simulink model "MVS_Dynamic_Trigger_Two_Layers_NoRA"  (R2024a)
settings: Solver=ode5  StartTime=0.0  StopTime=180  FixedStep=0.01  RelTol=1e-3
(part 2 of 4)

== system MVS_Dynamic_Trigger_Two_Layers_NoRA/High-Level Agent 1/Trajectory Planner ==
  e_tilde_xi : Inport
  e_tilde_vi : Inport  Port=2
  delta_xi : Inport  Port=3
  delta_vi : Inport  Port=4
  acc_ref : Inport  Port=5
  states_high : Inport  Port=6
  states_low : Inport  Port=7
  Achievability assurance : Subsystem
  Cooperative tracking : Subsystem
  Input compensator : MATLAB Function  TreatAsAtomicUnit=on
  State select : MATLAB Function  TreatAsAtomicUnit=on
  u_i : Outport
  wires:
  e_tilde_xi/1 -> Cooperative tracking/1(e_tilde_xi)
  e_tilde_vi/1 -> Cooperative tracking/2(e_tilde_vi)
  delta_xi/1 -> Cooperative tracking/3(delta_xi)
  delta_vi/1 -> Cooperative tracking/4(delta_vi)
  acc_ref/1 -> Cooperative tracking/5(acc_ref)
  Input compensator/1(u_i) -> u_i/1
  states_high/1 -> State select/1(states_high)
  states_low/1 -> State select/2(states_low)
  State select/1(v_i) -> Achievability assurance/1(v_i), Cooperative tracking/6(v_i)
  State select/2(delta_x_tilde) -> Achievability assurance/2(delta_x)
  State select/3(delta_v_tilde) -> Achievability assurance/3(delta_v)
  State select/4(a_d) -> Achievability assurance/4(a_d)
  Cooperative tracking/1(u_i_track) -> Input compensator/1(u_i_track)
  Achievability assurance/1(u_i_restrict) -> Input compensator/2(u_i_restrict)
  Achievability assurance/2(delta_low_norm) -> Input compensator/3(delta_low_norm)

== system MVS_Dynamic_Trigger_Two_Layers_NoRA/High-Level Agent 2/High-Level Dynamics ==
  u_i : Inport
  Memory : Memory  InitialCondition=zeros(3,1)
  Position : Integrator  InitialCondition=ini_pos
  Saturation_acc : Saturate  UpperLimit=acc_up_limit  LowerLimit=acc_low_limit
  Saturation_vel : Saturate  UpperLimit=vel_up_limit  LowerLimit=vel_low_limit
  Speed : Integrator  InitialCondition=[0;0;0]
  v_2 : Scope
  x_2 : Scope
  x_i : Outport
  v_i : Outport  Port=2
  a_i : Outport  Port=3
  wires:
  Position/1 -> x_i/1, x_2/1
  u_i/1 -> Memory/1
  Saturation_acc/1 -> a_i/1, Speed/1
  Speed/1 -> v_2/1, Saturation_vel/1
  Saturation_vel/1 -> v_i/1, Position/1
  Memory/1 -> Saturation_acc/1

== system MVS_Dynamic_Trigger_Two_Layers_NoRA/High-Level Agent 2/Trajectory Planner ==
  e_tilde_xi : Inport
  e_tilde_vi : Inport  Port=2
  delta_xi : Inport  Port=3
  delta_vi : Inport  Port=4
  acc_ref : Inport  Port=5
  states_high : Inport  Port=6
  states_low : Inport  Port=7
  Achievability assurance : Subsystem
  Cooperative tracking : Subsystem
  Input compensator : MATLAB Function  TreatAsAtomicUnit=on
  State select : MATLAB Function  TreatAsAtomicUnit=on
  u_i : Outport
  wires:
  e_tilde_xi/1 -> Cooperative tracking/1(e_tilde_xi)
  e_tilde_vi/1 -> Cooperative tracking/2(e_tilde_vi)
  delta_xi/1 -> Cooperative tracking/3(delta_xi)
  delta_vi/1 -> Cooperative tracking/4(delta_vi)
  acc_ref/1 -> Cooperative tracking/5(acc_ref)
  Input compensator/1(u_i) -> u_i/1
  states_high/1 -> State select/1(states_high)
  states_low/1 -> State select/2(states_low)
  State select/1(v_i) -> Achievability assurance/1(v_i), Cooperative tracking/6(v_i)
  State select/2(delta_x_tilde) -> Achievability assurance/2(delta_x)
  State select/3(delta_v_tilde) -> Achievability assurance/3(delta_v)
  State select/4(a_d) -> Achievability assurance/4(a_d)
  Cooperative tracking/1(u_i_track) -> Input compensator/1(u_i_track)
  Achievability assurance/1(u_i_restrict) -> Input compensator/2(u_i_restrict)
  Achievability assurance/2(delta_low_norm) -> Input compensator/3(delta_low_norm)

== system MVS_Dynamic_Trigger_Two_Layers_NoRA/High-Level Agent 3/High-Level Dynamics ==
  u_i : Inport
  Memory : Memory  InitialCondition=zeros(3,1)
  Position : Integrator  InitialCondition=ini_pos
  Saturation_acc : Saturate  UpperLimit=acc_up_limit  LowerLimit=acc_low_limit
  Saturation_vel : Saturate  UpperLimit=vel_up_limit  LowerLimit=vel_low_limit
  Speed : Integrator  InitialCondition=[0;0;0]
  v_3 : Scope
  x_3 : Scope
  x_i : Outport
  v_i : Outport  Port=2
  a_i : Outport  Port=3
  wires:
  Position/1 -> x_i/1, x_3/1
  u_i/1 -> Memory/1
  Saturation_acc/1 -> a_i/1, Speed/1
  Speed/1 -> v_3/1, Saturation_vel/1
  Saturation_vel/1 -> v_i/1, Position/1
  Memory/1 -> Saturation_acc/1

== system MVS_Dynamic_Trigger_Two_Layers_NoRA/High-Level Agent 3/Trajectory Planner ==
  e_tilde_xi : Inport
  e_tilde_vi : Inport  Port=2
  delta_xi : Inport  Port=3
  delta_vi : Inport  Port=4
  acc_ref : Inport  Port=5
  states_high : Inport  Port=6
  states_low : Inport  Port=7
  Achievability assurance : Subsystem
  Cooperative tracking : Subsystem
  Input compensator : MATLAB Function  TreatAsAtomicUnit=on
  State select : MATLAB Function  TreatAsAtomicUnit=on
  u_i : Outport
  wires:
  e_tilde_xi/1 -> Cooperative tracking/1(e_tilde_xi)
  e_tilde_vi/1 -> Cooperative tracking/2(e_tilde_vi)
  delta_xi/1 -> Cooperative tracking/3(delta_xi)
  delta_vi/1 -> Cooperative tracking/4(delta_vi)
  acc_ref/1 -> Cooperative tracking/5(acc_ref)
  Input compensator/1(u_i) -> u_i/1
  states_high/1 -> State select/1(states_high)
  states_low/1 -> State select/2(states_low)
  State select/1(v_i) -> Achievability assurance/1(v_i), Cooperative tracking/6(v_i)
  State select/2(delta_x_tilde) -> Achievability assurance/2(delta_x)
  State select/3(delta_v_tilde) -> Achievability assurance/3(delta_v)
  State select/4(a_d) -> Achievability assurance/4(a_d)
  Cooperative tracking/1(u_i_track) -> Input compensator/1(u_i_track)
  Achievability assurance/1(u_i_restrict) -> Input compensator/2(u_i_restrict)
  Achievability assurance/2(delta_low_norm) -> Input compensator/3(delta_low_norm)

== system MVS_Dynamic_Trigger_Two_Layers_NoRA/High-Level Agent 4/High-Level Dynamics ==
  u_i : Inport
  Memory : Memory  InitialCondition=zeros(3,1)
  Position : Integrator  InitialCondition=ini_pos
  Saturation_acc : Saturate  UpperLimit=acc_up_limit  LowerLimit=acc_low_limit
  Saturation_vel : Saturate  UpperLimit=vel_up_limit  LowerLimit=vel_low_limit
  Speed : Integrator  InitialCondition=[0;0;0]
  v_4 : Scope
  x_4 : Scope
  x_i : Outport
  v_i : Outport  Port=2
  a_i : Outport  Port=3
  wires:
  Position/1 -> x_i/1, x_4/1
  u_i/1 -> Memory/1
  Saturation_acc/1 -> a_i/1, Speed/1
  Speed/1 -> v_4/1, Saturation_vel/1
  Saturation_vel/1 -> v_i/1, Position/1
  Memory/1 -> Saturation_acc/1

== system MVS_Dynamic_Trigger_Two_Layers_NoRA/High-Level Agent 4/Trajectory Planner ==
  e_tilde_xi : Inport
  e_tilde_vi : Inport  Port=2
  delta_xi : Inport  Port=3
  delta_vi : Inport  Port=4
  acc_ref : Inport  Port=5
  states_high : Inport  Port=6
  states_low : Inport  Port=7
  Achievability assurance : Subsystem
  Cooperative tracking : Subsystem
  Input compensator : MATLAB Function  TreatAsAtomicUnit=on
  State select : MATLAB Function  TreatAsAtomicUnit=on
  u_i : Outport
  wires:
  e_tilde_xi/1 -> Cooperative tracking/1(e_tilde_xi)
  e_tilde_vi/1 -> Cooperative tracking/2(e_tilde_vi)
  delta_xi/1 -> Cooperative tracking/3(delta_xi)
  delta_vi/1 -> Cooperative tracking/4(delta_vi)
  acc_ref/1 -> Cooperative tracking/5(acc_ref)
  Input compensator/1(u_i) -> u_i/1
  states_high/1 -> State select/1(states_high)
  states_low/1 -> State select/2(states_low)
  State select/1(v_i) -> Achievability assurance/1(v_i), Cooperative tracking/6(v_i)
  State select/2(delta_x_tilde) -> Achievability assurance/2(delta_x)
  State select/3(delta_v_tilde) -> Achievability assurance/3(delta_v)
  State select/4(a_d) -> Achievability assurance/4(a_d)
  Cooperative tracking/1(u_i_track) -> Input compensator/1(u_i_track)
  Achievability assurance/1(u_i_restrict) -> Input compensator/2(u_i_restrict)
  Achievability assurance/2(delta_low_norm) -> Input compensator/3(delta_low_norm)

== system MVS_Dynamic_Trigger_Two_Layers_NoRA/High-Level Agent 5/High-Level Dynamics ==
  u_i : Inport
  Memory : Memory  InitialCondition=zeros(3,1)
  Position : Integrator  InitialCondition=ini_pos
  Saturation_acc : Saturate  UpperLimit=acc_up_limit  LowerLimit=acc_low_limit
  Saturation_vel : Saturate  UpperLimit=vel_up_limit  LowerLimit=vel_low_limit
  Speed : Integrator  InitialCondition=[0;0;0]
  v_5 : Scope
  x_5 : Scope
  x_i : Outport
  v_i : Outport  Port=2
  a_i : Outport  Port=3
  wires:
  Position/1 -> x_i/1, x_5/1
  u_i/1 -> Memory/1
  Saturation_acc/1 -> a_i/1, Speed/1
  Speed/1 -> v_5/1, Saturation_vel/1
  Saturation_vel/1 -> v_i/1, Position/1
  Memory/1 -> Saturation_acc/1

== system MVS_Dynamic_Trigger_Two_Layers_NoRA/High-Level Agent 5/Trajectory Planner ==
  e_tilde_xi : Inport
  e_tilde_vi : Inport  Port=2
  delta_xi : Inport  Port=3
  delta_vi : Inport  Port=4
  acc_ref : Inport  Port=5
  states_high : Inport  Port=6
  states_low : Inport  Port=7
  Achievability assurance : Subsystem
  Cooperative tracking : Subsystem
  Input compensator : MATLAB Function  TreatAsAtomicUnit=on
  State select : MATLAB Function  TreatAsAtomicUnit=on
  u_i : Outport
  wires:
  e_tilde_xi/1 -> Cooperative tracking/1(e_tilde_xi)
  e_tilde_vi/1 -> Cooperative tracking/2(e_tilde_vi)
  delta_xi/1 -> Cooperative tracking/3(delta_xi)
  delta_vi/1 -> Cooperative tracking/4(delta_vi)
  acc_ref/1 -> Cooperative tracking/5(acc_ref)
  Input compensator/1(u_i) -> u_i/1
  states_high/1 -> State select/1(states_high)
  states_low/1 -> State select/2(states_low)
  State select/1(v_i) -> Achievability assurance/1(v_i), Cooperative tracking/6(v_i)
  State select/2(delta_x_tilde) -> Achievability assurance/2(delta_x)
  State select/3(delta_v_tilde) -> Achievability assurance/3(delta_v)
  State select/4(a_d) -> Achievability assurance/4(a_d)
  Cooperative tracking/1(u_i_track) -> Input compensator/1(u_i_track)
  Achievability assurance/1(u_i_restrict) -> Input compensator/2(u_i_restrict)
  Achievability assurance/2(delta_low_norm) -> Input compensator/3(delta_low_norm)

== system MVS_Dynamic_Trigger_Two_Layers_NoRA/High-Level Agent 6/High-Level Dynamics ==
  u_i : Inport
  Memory : Memory  InitialCondition=zeros(3,1)
  Position : Integrator  InitialCondition=ini_pos
  Saturation_acc : Saturate  UpperLimit=acc_up_limit  LowerLimit=acc_low_limit
  Saturation_vel : Saturate  UpperLimit=vel_up_limit  LowerLimit=vel_low_limit
  Speed : Integrator  InitialCondition=[0;0;0]
  v_6 : Scope
  x_6 : Scope
  x_i : Outport
  v_i : Outport  Port=2
  a_i : Outport  Port=3
  wires:
  Position/1 -> x_i/1, x_6/1
  u_i/1 -> Memory/1
  Saturation_acc/1 -> a_i/1, Speed/1
  Speed/1 -> v_6/1, Saturation_vel/1
  Saturation_vel/1 -> v_i/1, Position/1
  Memory/1 -> Saturation_acc/1

== system MVS_Dynamic_Trigger_Two_Layers_NoRA/High-Level Agent 6/Trajectory Planner ==
  e_tilde_xi : Inport
  e_tilde_vi : Inport  Port=2
  delta_xi : Inport  Port=3
  delta_vi : Inport  Port=4
  acc_ref : Inport  Port=5
  states_high : Inport  Port=6
  states_low : Inport  Port=7
  Achievability assurance : Subsystem
  Cooperative tracking : Subsystem
  Input compensator : MATLAB Function  TreatAsAtomicUnit=on
  State select : MATLAB Function  TreatAsAtomicUnit=on
  u_i : Outport
  wires:
  e_tilde_xi/1 -> Cooperative tracking/1(e_tilde_xi)
  e_tilde_vi/1 -> Cooperative tracking/2(e_tilde_vi)
  delta_xi/1 -> Cooperative tracking/3(delta_xi)
  delta_vi/1 -> Cooperative tracking/4(delta_vi)
  acc_ref/1 -> Cooperative tracking/5(acc_ref)
  Input compensator/1(u_i) -> u_i/1
  states_high/1 -> State select/1(states_high)
  states_low/1 -> State select/2(states_low)
  State select/1(v_i) -> Achievability assurance/1(v_i), Cooperative tracking/6(v_i)
  State select/2(delta_x_tilde) -> Achievability assurance/2(delta_x)
  State select/3(delta_v_tilde) -> Achievability assurance/3(delta_v)
  State select/4(a_d) -> Achievability assurance/4(a_d)
  Cooperative tracking/1(u_i_track) -> Input compensator/1(u_i_track)
  Achievability assurance/1(u_i_restrict) -> Input compensator/2(u_i_restrict)
  Achievability assurance/2(delta_low_norm) -> Input compensator/3(delta_low_norm)

== system MVS_Dynamic_Trigger_Two_Layers_NoRA/UGV 1/Kinematics controller ==
  global_ref : Inport
  global_current_state : Inport  Port=2
  Body error : Scope
  Bus Creator : BusCreator  Inputs=2
  Clock : Clock
  Error calculation : MATLAB Function  TreatAsAtomicUnit=on
  Global error : Scope
  Saturation : Saturate  UpperLimit=[7; tan(2/9 * pi)]  LowerLimit=-[7; tan(2/9 * pi)]
  Control input : Outport
  wires:
  Bus Creator/1 -> Saturation/1
  Error calculation/1(vel_rear) -> Bus Creator/1
  global_ref/1 -> Error calculation/1(ref_3d)
  global_current_state/1 -> Error calculation/2(pos_bike)
  Error calculation/2(tan_sigma) -> Bus Creator/2
  Saturation/1 -> Control input/1
  Error calculation/3(pos_error_global) -> Global error/1
  Error calculation/4(pos_error_body) -> Body error/1
  Clock/1 -> Error calculation/3(t)

== system MVS_Dynamic_Trigger_Two_Layers_NoRA/UGV 2/Kinematics controller ==
  global_ref : Inport
  global_current_state : Inport  Port=2
  Body error : Scope
  Bus Creator : BusCreator  Inputs=2
  Clock : Clock
  Error calculation : MATLAB Function  TreatAsAtomicUnit=on
  Global error : Scope
  Saturation : Saturate  UpperLimit=[7; tan(2/9 * pi)]  LowerLimit=-[7; tan(2/9 * pi)]
  Control input : Outport
  wires:
  Bus Creator/1 -> Saturation/1
  Error calculation/1(vel_rear) -> Bus Creator/1
  global_ref/1 -> Error calculation/1(ref_3d)
  global_current_state/1 -> Error calculation/2(pos_bike)
  Error calculation/2(tan_sigma) -> Bus Creator/2
  Saturation/1 -> Control input/1
  Error calculation/3(pos_error_global) -> Global error/1
  Error calculation/4(pos_error_body) -> Body error/1
  Clock/1 -> Error calculation/3(t)

== system MVS_Dynamic_Trigger_Two_Layers_NoRA/UGV 3/Kinematics controller ==
  global_ref : Inport
  global_current_state : Inport  Port=2
  Body error : Scope
  Bus Creator : BusCreator  Inputs=2
  Error calculation : MATLAB Function  TreatAsAtomicUnit=on
  Global error : Scope
  Saturation : Saturate  UpperLimit=[7; tan(2/9 * pi)]  LowerLimit=-[7; tan(2/9 * pi)]
  Control input : Outport
  wires:
  Bus Creator/1 -> Saturation/1
  Error calculation/1(vel_rear) -> Bus Creator/1
  global_ref/1 -> Error calculation/1(ref_3d)
  global_current_state/1 -> Error calculation/2(pos_bike)
  Error calculation/2(tan_sigma) -> Bus Creator/2
  Saturation/1 -> Control input/1
  Error calculation/3(pos_error_global) -> Global error/1
  Error calculation/4(pos_error_body) -> Body error/1

== system MVS_Dynamic_Trigger_Two_Layers_NoRA/UGV 4/Kinematics controller ==
  global_ref : Inport
  global_current_state : Inport  Port=2
  Body error : Scope
  Bus Creator : BusCreator  Inputs=2
  Error calculation : MATLAB Function  TreatAsAtomicUnit=on
  Global error : Scope
  Saturation : Saturate  UpperLimit=[7; tan(2/9 * pi)]  LowerLimit=-[7; tan(2/9 * pi)]
  Control input : Outport
  wires:
  Bus Creator/1 -> Saturation/1
  Error calculation/1(vel_rear) -> Bus Creator/1
  global_ref/1 -> Error calculation/1(ref_3d)
  global_current_state/1 -> Error calculation/2(pos_bike)
  Error calculation/2(tan_sigma) -> Bus Creator/2
  Saturation/1 -> Control input/1
  Error calculation/3(pos_error_global) -> Global error/1
  Error calculation/4(pos_error_body) -> Body error/1

== system MVS_Dynamic_Trigger_Two_Layers_NoRA/Communication Preparation 1/Reference Filter/Adaptive filter ==
  pos_ref : Inport
  vel_ref : Inport  Port=2
  current_pos : Inport  Port=3
  Filter error 1 : Scope
  Input compensator : MATLAB Function  TreatAsAtomicUnit=on
  Integrator : Integrator  InitialCondition=[0;0;0]
  Nominal filter : MATLAB Function  TreatAsAtomicUnit=on
  Scope : Scope
  u_i : Outport
  filter_error : Outport  Port=2
  wires:
  current_pos/1 -> Nominal filter/3(current_pos)
  vel_ref/1 -> Nominal filter/2(vel_ref)
  pos_ref/1 -> Nominal filter/1(pos_ref)
  Nominal filter/1(u_i_nom) -> Input compensator/1(u_i_nom)
  Input compensator/2(Xi_i_dot) -> Integrator/1
  Integrator/1 -> Scope/1, Input compensator/2(Xi_i)
  Input compensator/1(u_i) -> u_i/1
  Nominal filter/2(filter_error) -> filter_error/1, Filter error 1/1

== system MVS_Dynamic_Trigger_Two_Layers_NoRA/Communication Preparation 2/Reference Filter/Adaptive filter ==
  pos_ref : Inport
  vel_ref : Inport  Port=2
  current_pos : Inport  Port=3
  Filter error 2 : Scope
  Input compensator : MATLAB Function  TreatAsAtomicUnit=on
  Integrator : Integrator  InitialCondition=[0;0;0]
  Nominal filter : MATLAB Function  TreatAsAtomicUnit=on
  Xi_filter_2 : Scope
  u_i : Outport
  filter_error : Outport  Port=2
  wires:
  current_pos/1 -> Nominal filter/3(current_pos)
  vel_ref/1 -> Nominal filter/2(vel_ref)
  pos_ref/1 -> Nominal filter/1(pos_ref)
  Nominal filter/1(u_i_nom) -> Input compensator/1(u_i_nom)
  Input compensator/2(Xi_i_dot) -> Integrator/1
  Integrator/1 -> Xi_filter_2/1, Input compensator/2(Xi_i)
  Input compensator/1(u_i) -> u_i/1
  Nominal filter/2(filter_error) -> filter_error/1, Filter error 2/1

== system MVS_Dynamic_Trigger_Two_Layers_NoRA/Communication Preparation 3/Reference Filter/Adaptive filter ==
  pos_ref : Inport
  vel_ref : Inport  Port=2
  current_pos : Inport  Port=3
  Filter error 3 : Scope
  Input compensator : MATLAB Function  TreatAsAtomicUnit=on
  Integrator : Integrator  InitialCondition=[0;0;0]
  Nominal filter : MATLAB Function  TreatAsAtomicUnit=on
  Xi_filter_3 : Scope
  u_i : Outport
  filter_error : Outport  Port=2
  wires:
  current_pos/1 -> Nominal filter/3(current_pos)
  vel_ref/1 -> Nominal filter/2(vel_ref)
  pos_ref/1 -> Nominal filter/1(pos_ref)
  Nominal filter/1(u_i_nom) -> Input compensator/1(u_i_nom)
  Input compensator/2(Xi_i_dot) -> Integrator/1
  Integrator/1 -> Xi_filter_3/1, Input compensator/2(Xi_i)
  Input compensator/1(u_i) -> u_i/1
  Nominal filter/2(filter_error) -> filter_error/1, Filter error 3/1

== system MVS_Dynamic_Trigger_Two_Layers_NoRA/Communication Preparation 4/Reference Filter/Adaptive filter ==
  pos_ref : Inport
  vel_ref : Inport  Port=2
  current_pos : Inport  Port=3
  Filter error 4 : Scope
  Input compensator : MATLAB Function  TreatAsAtomicUnit=on
  Integrator : Integrator  InitialCondition=[0;0;0]
  Nominal filter : MATLAB Function  TreatAsAtomicUnit=on
  Xi_filter_4 : Scope
  u_i : Outport
  filter_error : Outport  Port=2
  wires:
  current_pos/1 -> Nominal filter/3(current_pos)
  vel_ref/1 -> Nominal filter/2(vel_ref)
  pos_ref/1 -> Nominal filter/1(pos_ref)
  Nominal filter/1(u_i_nom) -> Input compensator/1(u_i_nom)
  Input compensator/2(Xi_i_dot) -> Integrator/1
  Integrator/1 -> Xi_filter_4/1, Input compensator/2(Xi_i)
  Input compensator/1(u_i) -> u_i/1
  Nominal filter/2(filter_error) -> filter_error/1, Filter error 4/1

== system MVS_Dynamic_Trigger_Two_Layers_NoRA/Communication Preparation 5/Reference Filter/Adaptive filter ==
  pos_ref : Inport
  vel_ref : Inport  Port=2
  current_pos : Inport  Port=3
  Filter error 5 : Scope
  Input compensator : MATLAB Function  TreatAsAtomicUnit=on
  Integrator : Integrator  InitialCondition=[0;0;0]
  Nominal filter : MATLAB Function  TreatAsAtomicUnit=on
  Xi_filter_5 : Scope
  u_i : Outport
  filter_error : Outport  Port=2
  wires:
  current_pos/1 -> Nominal filter/3(current_pos)
  vel_ref/1 -> Nominal filter/2(vel_ref)
  pos_ref/1 -> Nominal filter/1(pos_ref)
  Nominal filter/1(u_i_nom) -> Input compensator/1(u_i_nom)
  Input compensator/2(Xi_i_dot) -> Integrator/1
  Integrator/1 -> Xi_filter_5/1, Input compensator/2(Xi_i)
  Input compensator/1(u_i) -> u_i/1
  Nominal filter/2(filter_error) -> filter_error/1, Filter error 5/1

== system MVS_Dynamic_Trigger_Two_Layers_NoRA/Communication Preparation 6/Reference Filter/Adaptive filter ==
  pos_ref : Inport
  vel_ref : Inport  Port=2
  current_pos : Inport  Port=3
  Filter error 6 : Scope
  Input compensator : MATLAB Function  TreatAsAtomicUnit=on
  Integrator : Integrator  InitialCondition=[0;0;0]
  Nominal filter : MATLAB Function  TreatAsAtomicUnit=on
  Xi_filter_6 : Scope
  u_i : Outport
  filter_error : Outport  Port=2
  wires:
  current_pos/1 -> Nominal filter/3(current_pos)
  vel_ref/1 -> Nominal filter/2(vel_ref)
  pos_ref/1 -> Nominal filter/1(pos_ref)
  Nominal filter/1(u_i_nom) -> Input compensator/1(u_i_nom)
  Input compensator/2(Xi_i_dot) -> Integrator/1
  Integrator/1 -> Xi_filter_6/1, Input compensator/2(Xi_i)
  Input compensator/1(u_i) -> u_i/1
  Nominal filter/2(filter_error) -> filter_error/1, Filter error 6/1

== system MVS_Dynamic_Trigger_Two_Layers_NoRA/High-Level Agent 1/Trajectory Planner/Achievability assurance ==
  v_i : Inport
  delta_x : Inport  Port=2
  delta_v : Inport  Port=3
  a_d : Inport  Port=4
  Input compensator : MATLAB Function  TreatAsAtomicUnit=on
  Integrator : Integrator  InitialCondition=[0;0;0]
  Nominal SMC : MATLAB Function  TreatAsAtomicUnit=on
  low_error_norm_1 : Scope
  u_i_res : Scope
  u_i_restrict : Outport
  delta_low_norm : Outport  Port=2
  wires:
  delta_x/1 -> Nominal SMC/1(delta_x)
  delta_v/1 -> Nominal SMC/2(delta_v)
  a_d/1 -> Nominal SMC/3(a_d)
  Nominal SMC/2(delta_norm) -> delta_low_norm/1, low_error_norm_1/1
  Integrator/1 -> Input compensator/3(Xi_i)
  Input compensator/2(Xi_i_dot) -> Integrator/1
  Input compensator/1(u_i_actual) -> u_i_res/1, u_i_restrict/1
  v_i/1 -> Input compensator/2(v_i)
  Nominal SMC/1(u_restrict) -> Input compensator/1(u_i_restrict)

== system MVS_Dynamic_Trigger_Two_Layers_NoRA/High-Level Agent 1/Trajectory Planner/Cooperative tracking ==
  e_tilde_xi : Inport
  e_tilde_vi : Inport  Port=2
  delta_xi : Inport  Port=3
  delta_vi : Inport  Port=4
  acc_ref : Inport  Port=5
  v_i : Inport  Port=6
  Input compensator : MATLAB Function  TreatAsAtomicUnit=on
  Integrator : Integrator  InitialCondition=[0;0;0]
  Nominal sliding mode controller : MATLAB Function  TreatAsAtomicUnit=on
  u_i_tra : Scope
  u_i_track : Outport
  wires:
  acc_ref/1 -> Nominal sliding mode controller/5(acl_ref_agent)
  Input compensator/1(u_i_actual) -> u_i_tra/1, u_i_track/1
  Nominal sliding mode controller/1(u_i_slide) -> Input compensator/1(u_i_slide)
  e_tilde_vi/1 -> Nominal sliding mode controller/2(e_tilde_vi)
  v_i/1 -> Input compensator/2(v_i)
  delta_xi/1 -> Nominal sliding mode controller/3(delta_xi)
  delta_vi/1 -> Nominal sliding mode controller/4(delta_vi)
  e_tilde_xi/1 -> Nominal sliding mode controller/1(e_tilde_xi)
  Input compensator/2(Xi_i_dot) -> Integrator/1
  Integrator/1 -> Input compensator/3(Xi_i)

== system MVS_Dynamic_Trigger_Two_Layers_NoRA/High-Level Agent 2/Trajectory Planner/Achievability assurance ==
  v_i : Inport
  delta_x : Inport  Port=2
  delta_v : Inport  Port=3
  a_d : Inport  Port=4
  Input compensator : MATLAB Function  TreatAsAtomicUnit=on
  Integrator : Integrator  InitialCondition=[0;0;0]
  Nominal SMC : MATLAB Function  TreatAsAtomicUnit=on
  low_error_norm_2 : Scope
  u_i_res : Scope
  u_i_restrict : Outport
  delta_low_norm : Outport  Port=2
  wires:
  delta_x/1 -> Nominal SMC/1(delta_x)
  delta_v/1 -> Nominal SMC/2(delta_v)
  a_d/1 -> Nominal SMC/3(a_d)
  Nominal SMC/2(delta_norm) -> delta_low_norm/1, low_error_norm_2/1
  Integrator/1 -> Input compensator/3(Xi_i)
  Input compensator/2(Xi_i_dot) -> Integrator/1
  Input compensator/1(u_i_actual) -> u_i_res/1, u_i_restrict/1
  v_i/1 -> Input compensator/2(v_i)
  Nominal SMC/1(u_restrict) -> Input compensator/1(u_i_restrict)

== system MVS_Dynamic_Trigger_Two_Layers_NoRA/High-Level Agent 2/Trajectory Planner/Cooperative tracking ==
  e_tilde_xi : Inport
  e_tilde_vi : Inport  Port=2
  delta_xi : Inport  Port=3
  delta_vi : Inport  Port=4
  acc_ref : Inport  Port=5
  v_i : Inport  Port=6
  Input compensator : MATLAB Function  TreatAsAtomicUnit=on
  Integrator : Integrator  InitialCondition=[0;0;0]
  Nominal sliding mode controller : MATLAB Function  TreatAsAtomicUnit=on
  u_i_tra : Scope
  u_i_track : Outport
  wires:
  acc_ref/1 -> Nominal sliding mode controller/5(acl_ref_agent)
  Input compensator/1(u_i_actual) -> u_i_tra/1, u_i_track/1
  Nominal sliding mode controller/1(u_i_slide) -> Input compensator/1(u_i_slide)
  e_tilde_vi/1 -> Nominal sliding mode controller/2(e_tilde_vi)
  v_i/1 -> Input compensator/2(v_i)
  delta_xi/1 -> Nominal sliding mode controller/3(delta_xi)
  delta_vi/1 -> Nominal sliding mode controller/4(delta_vi)
  e_tilde_xi/1 -> Nominal sliding mode controller/1(e_tilde_xi)
  Input compensator/2(Xi_i_dot) -> Integrator/1
  Integrator/1 -> Input compensator/3(Xi_i)

== system MVS_Dynamic_Trigger_Two_Layers_NoRA/High-Level Agent 3/Trajectory Planner/Achievability assurance ==
  v_i : Inport
  delta_x : Inport  Port=2
  delta_v : Inport  Port=3
  a_d : Inport  Port=4
  Input compensator : MATLAB Function  TreatAsAtomicUnit=on
  Integrator : Integrator  InitialCondition=[0;0;0]
  Nominal SMC : MATLAB Function  TreatAsAtomicUnit=on
  low_error_norm_3 : Scope
  u_i_res : Scope
  u_i_restrict : Outport
  delta_low_norm : Outport  Port=2
  wires:
  delta_x/1 -> Nominal SMC/1(delta_x)
  delta_v/1 -> Nominal SMC/2(delta_v)
  a_d/1 -> Nominal SMC/3(a_d)
  Nominal SMC/2(delta_norm) -> delta_low_norm/1, low_error_norm_3/1
  Integrator/1 -> Input compensator/3(Xi_i)
  Input compensator/2(Xi_i_dot) -> Integrator/1
  Input compensator/1(u_i_actual) -> u_i_res/1, u_i_restrict/1
  v_i/1 -> Input compensator/2(v_i)
  Nominal SMC/1(u_restrict) -> Input compensator/1(u_i_restrict)

== system MVS_Dynamic_Trigger_Two_Layers_NoRA/High-Level Agent 3/Trajectory Planner/Cooperative tracking ==
  e_tilde_xi : Inport
  e_tilde_vi : Inport  Port=2
  delta_xi : Inport  Port=3
  delta_vi : Inport  Port=4
  acc_ref : Inport  Port=5
  v_i : Inport  Port=6
  Input compensator : MATLAB Function  TreatAsAtomicUnit=on
  Integrator : Integrator  InitialCondition=[0;0;0]
  Nominal sliding mode controller : MATLAB Function  TreatAsAtomicUnit=on
  u_i_tra : Scope
  u_i_track : Outport
  wires:
  acc_ref/1 -> Nominal sliding mode controller/5(acl_ref_agent)
  Input compensator/1(u_i_actual) -> u_i_tra/1, u_i_track/1
  Nominal sliding mode controller/1(u_i_slide) -> Input compensator/1(u_i_slide)
  e_tilde_vi/1 -> Nominal sliding mode controller/2(e_tilde_vi)
  v_i/1 -> Input compensator/2(v_i)
  delta_xi/1 -> Nominal sliding mode controller/3(delta_xi)
  delta_vi/1 -> Nominal sliding mode controller/4(delta_vi)
  e_tilde_xi/1 -> Nominal sliding mode controller/1(e_tilde_xi)
  Input compensator/2(Xi_i_dot) -> Integrator/1
  Integrator/1 -> Input compensator/3(Xi_i)

== system MVS_Dynamic_Trigger_Two_Layers_NoRA/High-Level Agent 4/Trajectory Planner/Achievability assurance ==
  v_i : Inport
  delta_x : Inport  Port=2
  delta_v : Inport  Port=3
  a_d : Inport  Port=4
  Input compensator : MATLAB Function  TreatAsAtomicUnit=on
  Integrator : Integrator  InitialCondition=[0;0;0]
  Nominal SMC : MATLAB Function  TreatAsAtomicUnit=on
  low_error_norm_4 : Scope
  u_i_res : Scope
  u_i_restrict : Outport
  delta_low_norm : Outport  Port=2
  wires:
  delta_x/1 -> Nominal SMC/1(delta_x)
  delta_v/1 -> Nominal SMC/2(delta_v)
  a_d/1 -> Nominal SMC/3(a_d)
  Nominal SMC/2(delta_norm) -> delta_low_norm/1, low_error_norm_4/1
  Integrator/1 -> Input compensator/3(Xi_i)
  Input compensator/2(Xi_i_dot) -> Integrator/1
  Input compensator/1(u_i_actual) -> u_i_res/1, u_i_restrict/1
  v_i/1 -> Input compensator/2(v_i)
  Nominal SMC/1(u_restrict) -> Input compensator/1(u_i_restrict)

== system MVS_Dynamic_Trigger_Two_Layers_NoRA/High-Level Agent 4/Trajectory Planner/Cooperative tracking ==
  e_tilde_xi : Inport
  e_tilde_vi : Inport  Port=2
  delta_xi : Inport  Port=3
  delta_vi : Inport  Port=4
  acc_ref : Inport  Port=5
  v_i : Inport  Port=6
  Input compensator : MATLAB Function  TreatAsAtomicUnit=on
  Integrator : Integrator  InitialCondition=[0;0;0]
  Nominal sliding mode controller : MATLAB Function  TreatAsAtomicUnit=on
  u_i_tra : Scope
  u_i_track : Outport
  wires:
  acc_ref/1 -> Nominal sliding mode controller/5(acl_ref_agent)
  Input compensator/1(u_i_actual) -> u_i_tra/1, u_i_track/1
  Nominal sliding mode controller/1(u_i_slide) -> Input compensator/1(u_i_slide)
  e_tilde_vi/1 -> Nominal sliding mode controller/2(e_tilde_vi)
  v_i/1 -> Input compensator/2(v_i)
  delta_xi/1 -> Nominal sliding mode controller/3(delta_xi)
  delta_vi/1 -> Nominal sliding mode controller/4(delta_vi)
  e_tilde_xi/1 -> Nominal sliding mode controller/1(e_tilde_xi)
  Input compensator/2(Xi_i_dot) -> Integrator/1
  Integrator/1 -> Input compensator/3(Xi_i)

== system MVS_Dynamic_Trigger_Two_Layers_NoRA/High-Level Agent 5/Trajectory Planner/Achievability assurance ==
  v_i : Inport
  delta_x : Inport  Port=2
  delta_v : Inport  Port=3
  a_d : Inport  Port=4
  Input compensator : MATLAB Function  TreatAsAtomicUnit=on
  Integrator : Integrator  InitialCondition=[0;0;0]
  Nominal SMC : MATLAB Function  TreatAsAtomicUnit=on
  low_error_norm_5 : Scope
  u_i_res : Scope
  u_i_restrict : Outport
  delta_low_norm : Outport  Port=2
  wires:
  delta_x/1 -> Nominal SMC/1(delta_x)
  delta_v/1 -> Nominal SMC/2(delta_v)
  a_d/1 -> Nominal SMC/3(a_d)
  Nominal SMC/2(delta_norm) -> delta_low_norm/1, low_error_norm_5/1
  Integrator/1 -> Input compensator/3(Xi_i)
  Input compensator/2(Xi_i_dot) -> Integrator/1
  Input compensator/1(u_i_actual) -> u_i_res/1, u_i_restrict/1
  v_i/1 -> Input compensator/2(v_i)
  Nominal SMC/1(u_restrict) -> Input compensator/1(u_i_restrict)

== system MVS_Dynamic_Trigger_Two_Layers_NoRA/High-Level Agent 5/Trajectory Planner/Cooperative tracking ==
  e_tilde_xi : Inport
  e_tilde_vi : Inport  Port=2
  delta_xi : Inport  Port=3
  delta_vi : Inport  Port=4
  acc_ref : Inport  Port=5
  v_i : Inport  Port=6
  Input compensator : MATLAB Function  TreatAsAtomicUnit=on
  Integrator : Integrator  InitialCondition=[0;0;0]
  Nominal sliding mode controller : MATLAB Function  TreatAsAtomicUnit=on
  u_i_tra : Scope
  u_i_track : Outport
  wires:
  acc_ref/1 -> Nominal sliding mode controller/5(acl_ref_agent)
  Input compensator/1(u_i_actual) -> u_i_tra/1, u_i_track/1
  Nominal sliding mode controller/1(u_i_slide) -> Input compensator/1(u_i_slide)
  e_tilde_vi/1 -> Nominal sliding mode controller/2(e_tilde_vi)
  v_i/1 -> Input compensator/2(v_i)
  delta_xi/1 -> Nominal sliding mode controller/3(delta_xi)
  delta_vi/1 -> Nominal sliding mode controller/4(delta_vi)
  e_tilde_xi/1 -> Nominal sliding mode controller/1(e_tilde_xi)
  Input compensator/2(Xi_i_dot) -> Integrator/1
  Integrator/1 -> Input compensator/3(Xi_i)

== system MVS_Dynamic_Trigger_Two_Layers_NoRA/High-Level Agent 6/Trajectory Planner/Achievability assurance ==
  v_i : Inport
  delta_x : Inport  Port=2
  delta_v : Inport  Port=3
  a_d : Inport  Port=4
  Input compensator : MATLAB Function  TreatAsAtomicUnit=on
  Integrator : Integrator  InitialCondition=[0;0;0]
  Nominal SMC : MATLAB Function  TreatAsAtomicUnit=on
  low_error_norm_6 : Scope
  u_i_res : Scope
  u_i_restrict : Outport
  delta_low_norm : Outport  Port=2
  wires:
  delta_x/1 -> Nominal SMC/1(delta_x)
  delta_v/1 -> Nominal SMC/2(delta_v)
  a_d/1 -> Nominal SMC/3(a_d)
  Nominal SMC/2(delta_norm) -> delta_low_norm/1, low_error_norm_6/1
  Integrator/1 -> Input compensator/3(Xi_i)
  Input compensator/2(Xi_i_dot) -> Integrator/1
  Input compensator/1(u_i_actual) -> u_i_res/1, u_i_restrict/1
  v_i/1 -> Input compensator/2(v_i)
  Nominal SMC/1(u_restrict) -> Input compensator/1(u_i_restrict)

== system MVS_Dynamic_Trigger_Two_Layers_NoRA/High-Level Agent 6/Trajectory Planner/Cooperative tracking ==
  e_tilde_xi : Inport
  e_tilde_vi : Inport  Port=2
  delta_xi : Inport  Port=3
  delta_vi : Inport  Port=4
  acc_ref : Inport  Port=5
  v_i : Inport  Port=6
  Input compensator : MATLAB Function  TreatAsAtomicUnit=on
  Integrator : Integrator  InitialCondition=[0;0;0]
  Nominal sliding mode controller : MATLAB Function  TreatAsAtomicUnit=on
  u_i_tra : Scope
  u_i_track : Outport
  wires:
  acc_ref/1 -> Nominal sliding mode controller/5(acl_ref_agent)
  Input compensator/1(u_i_actual) -> u_i_tra/1, u_i_track/1
  Nominal sliding mode controller/1(u_i_slide) -> Input compensator/1(u_i_slide)
  e_tilde_vi/1 -> Nominal sliding mode controller/2(e_tilde_vi)
  v_i/1 -> Input compensator/2(v_i)
  delta_xi/1 -> Nominal sliding mode controller/3(delta_xi)
  delta_vi/1 -> Nominal sliding mode controller/4(delta_vi)
  e_tilde_xi/1 -> Nominal sliding mode controller/1(e_tilde_xi)
  Input compensator/2(Xi_i_dot) -> Integrator/1
  Integrator/1 -> Input compensator/3(Xi_i)

== matlab function MVS_Dynamic_Trigger_Two_Layers_NoRA/AAV 2/Plant ==
  data: x_ddot output; w_i output; state_all input; u_i input; t input
function [x_ddot, w_i] = model(state_all, u_i, t)

%% Second-order plants for robots
dimension = 3;
serial_num = 6;
v_i = state_all(dimension * 1 + 1: dimension * 2);

K_i = 0.1 * [1;1;1];
m_i = 5;
g = 9.81;

f_i = -[K_i(1) * v_i(1) / m_i; K_i(2) * v_i(2) /m_i; K_i(3) * v_i(3)/ m_i + g];

if t >= 110 && t <= 125 
    w_i = [-1.2 * cos(0.5 * t - serial_num * pi/2); 0.7 * sin(0.4 * t + serial_num * pi/3); 1.1 * sin(0.6 * t + serial_num * pi/4)];
else
    w_i = zeros(3,1);
end

x_ddot = f_i + u_i + w_i;

end

== matlab function MVS_Dynamic_Trigger_Two_Layers_NoRA/AAV 2/Reference_abstract ==
  data: a_di output; ref input; state_all input; delta_xi output; delta_vi output
function [a_di, delta_xi, delta_vi] = ref_obtain(ref, state_all)

%% Basic parameters

dimension = 3;

x_i = state_all(dimension * 0 + 1: dimension * 1);
v_i = state_all(dimension * 1 + 1: dimension * 2);

x_di = ref(dimension * 0 + 1: dimension * 1);
v_di = ref(dimension * 1 + 1: dimension * 2);
a_di = ref(dimension * 2 + 1: dimension * 3);

delta_xi = x_i - x_di; 
delta_vi = v_i - v_di;

end

== matlab function MVS_Dynamic_Trigger_Two_Layers_NoRA/AAV 1/Controller/MATLAB Function ==
  data: u_nom input; u_diff output; u_sat input
function u_diff = fcn(u_nom, u_sat)

u_diff = norm(u_nom - u_sat);

end

== matlab function MVS_Dynamic_Trigger_Two_Layers_NoRA/Laplacian info/Communication topology ==
  data: L output
function L = commu_topology()

% L = [4, -1, 0, -1, -1, -1;
%      -1, 2, 0, 0, -1, 0;
%      0, 0, 1, -1, 0, 0;
%      -1, 0, -1, 3, -1, 0;
%      0, -1, 0, 0, 2, -1;
%      0, 0, 0, 0, -1, 1];

L = [3, -1, 0, -1, 0, -1;
     -1, 3, -1, 0, -1, 0;
     0, -1, 2, -1, 0, 0;
     -1, 0, -1, 3, 0, -1;
     -1, 0, 0, 0, 2, -1;
     0, 0, 0, 0, -1, 1];

end

== matlab function MVS_Dynamic_Trigger_Two_Layers_NoRA/Communication Preparation 3/Reference Filter/Adaptive filter/Input compensator ==
  data: u_i_nom input; u_i output; Xi_i input; Xi_i_dot output
function [u_i, Xi_i_dot] = input_compensator(u_i_nom, Xi_i)

%% Basic parameters
eta_1 = 10 * eye(3);
eta_2 = 0.5 * eye(3);
eta_3 = 6 * eye(3);
v_Mi = [5;5;4];

Xi_m = 5;

%% Calculate the actual control input
u_i = u_i_nom - eta_3 * Xi_i;
u_i_actual = u_i;

u_up = v_Mi;
u_low = - v_Mi;

for i = 1 : size(u_i_actual,1)
    if u_i(i) > u_up(i)
        u_i_actual(i) = u_up(i);
    elseif u_i(i) < u_low(i)
        u_i_actual(i) = u_low(i);
    end
end

u_tilde_i = u_i - u_i_actual;

if norm(Xi_i) < Xi_m
    Xi_i_dot = eta_1 * u_tilde_i - eta_2 * Xi_i;
else
    Xi_i_dot = eta_1 * u_tilde_i - eta_2 * Xi_i - norm(u_tilde_i)^2/norm(Xi_i)^2;
end

% Xi_i_dot = [0;0;0];

end

== matlab function MVS_Dynamic_Trigger_Two_Layers_NoRA/High-Level Agent 3/Information receiver ==
  data: e_tilde_xi output; info_indi input; info_all input; e_tilde_vi output; delta_xi output; delta_vi output; acl_ref_agent output; Laplacian input
function [e_tilde_xi, e_tilde_vi, delta_xi, delta_vi, acl_ref_agent] = info_selector(info_indi, info_all, Laplacian)

%% Notation
% info_indi = [delta_xi, delta_vi, v_d_dot]
% info_all is the info obtained from event triggered communication, note
% that we cannot use this directly because each agent should know its own
% tracking errors
% Laplacian is the Laplacian matrix of the communication topology

%% Basic parameters
serial_num = 3;
dimension = 3;

%% Information selection
L_i = kron(Laplacian(serial_num, :), eye(3));
num_agent = size(Laplacian, 1);

% Current agent states
delta_xi = info_indi(1:3);
delta_vi = info_indi(4:6);
acl_ref_agent = info_indi(7:9);

% Select position error and the velocity error
delta_x_all = kron(eye(num_agent), [eye(dimension), zeros(dimension)]) * info_all;
delta_v_all = kron(eye(num_agent), [zeros(dimension), eye(dimension)]) * info_all;

% Replace the event-triggered error with its own real-time errors
delta_x_all( (serial_num - 1) * dimension + 1: serial_num * dimension ) = delta_xi;
delta_v_all( (serial_num - 1) * dimension + 1: serial_num * dimension ) = delta_vi;

% Calculate the cooperative errors
e_tilde_xi = L_i * delta_x_all;
e_tilde_vi = L_i * delta_v_all;

end

== matlab function MVS_Dynamic_Trigger_Two_Layers_NoRA/High-Level Agent 3/Trajectory Planner/Achievability assurance/Input compensator ==
  data: u_i_restrict input; v_i input; u_i_actual output; Xi_i input; Xi_i_dot output
function [u_i_actual, Xi_i_dot] = input_compensator(u_i_restrict, v_i, Xi_i)

%% Basic parameters
eta_1 = 10 * eye(3);
eta_2 = 0.5 * eye(3);
eta_3 = 6 * eye(3);
U_Mi = [2;2;1.5];

Xi_m = 5;

%% Preliminary compensation
v_Mi = [5;5;4];
control_step = 0.01;
v_up = v_Mi - v_i;
v_low = -v_Mi - v_i;
u_up = min(v_up/control_step, U_Mi);
u_low = max(v_low/control_step, -U_Mi);

%% Calculate the actual control input
u_i = u_i_restrict - eta_3 * Xi_i;
u_i_actual = u_i;

for i = 1 : size(u_i_actual,1)
    if u_i(i) > u_up(i)
        u_i_actual(i) = u_up(i);
    elseif u_i(i) < u_low(i)
        u_i_actual(i) = u_low(i);
    end
end

u_tilde_i = u_i - u_i_actual;

if norm(Xi_i) < Xi_m
    Xi_i_dot = eta_1 * u_tilde_i - eta_2 * Xi_i;
else
    Xi_i_dot = eta_1 * u_tilde_i - eta_2 * Xi_i - norm(u_tilde_i)^2/norm(Xi_i)^2;
end

end

== matlab function MVS_Dynamic_Trigger_Two_Layers_NoRA/High-Level Agent 3/Trajectory Planner/Achievability assurance/Nominal SMC ==
  data: delta_x input; u_restrict output; delta_v input; a_d input; delta_norm output
function [u_restrict, delta_norm] = slide_control(delta_x, delta_v, a_d)

c = 1 * eye(3);
lambda = 1 * eye(3);
r_1 = 1.5;        % Maximum difference
% r_2 = 0.5;
k_tilde = 2;

s = delta_v + lambda * delta_x;
delta_norm = norm(delta_x);

choice = 1;

switch choice
    case 1
        u_restrict = a_d - lambda * delta_v - c * s - k_tilde /(r_1^2 - norm(delta_x)^2) * delta_x;
    case 2
        u_restrict = a_d - lambda * delta_v - c * s - delta_x;
    case 3
        u_restrict = - lambda * delta_v - c * s - k_tilde * 3 * delta_x / (r_1^2 - norm(delta_x)^2);
    case 4
        u_restrict = - lambda * delta_v - c * s - k_tilde * delta_x;
end

%% Known physical acceleration
% u_restrict = a_d - lambda * delta_v - (r_1^2 - norm(s)^2) * c * s;
% u_restrict = a_d - lambda * delta_v - c * s - 2 * max(3 /(r_1^2 - norm(delta_x)^2), 1) * delta_x;
% u_restrict = a_d - lambda * delta_v - c * s - 2 * (r_1^2 - r_2^2) /(r_1^2 - norm(delta_x)^2) * delta_x;
% u_restrict = a_d - lambda * delta_v - c * s - delta_x;

%% Unknown physical acceleration
% u_restrict = - lambda * delta_v - c * s - 2 * 3 * delta_x / (r_1^2 - norm(delta_x)^2);
% u_restrict = - lambda * delta_v - c * s - 2 * delta_x;

end

== matlab function MVS_Dynamic_Trigger_Two_Layers_NoRA/High-Level Agent 3/Trajectory Planner/Cooperative tracking/Input compensator ==
  data: u_i_slide input; v_i input; u_i_actual output; Xi_i input; Xi_i_dot output
function [u_i_actual, Xi_i_dot] = input_compensator(u_i_slide, v_i, Xi_i)

%% Basic parameters
eta_1 = 10 * eye(3);
eta_2 = 0.5 * eye(3);
eta_3 = 6 * eye(3);
U_Mi = [2;2;1.5];

Xi_m = 5;

%% Preliminary compensation
v_Mi = [5;5;4];
control_step = 0.01;
v_up = v_Mi - v_i;
v_low = -v_Mi - v_i;
u_up = min(v_up/control_step, U_Mi);
u_low = max(v_low/control_step, -U_Mi);

%% Calculate the actual control input
u_i = u_i_slide - eta_3 * Xi_i;
u_i_actual = u_i;

for i = 1 : size(u_i_actual,1)
    if u_i(i) > u_up(i)
        u_i_actual(i) = u_up(i);
    elseif u_i(i) < u_low(i)
        u_i_actual(i) = u_low(i);
    end
end

u_tilde_i = u_i - u_i_actual;

if norm(Xi_i) < Xi_m
    Xi_i_dot = eta_1 * u_tilde_i - eta_2 * Xi_i;
else
    Xi_i_dot = eta_1 * u_tilde_i - eta_2 * Xi_i - norm(u_tilde_i)^2/norm(Xi_i)^2;
end

end

== matlab function MVS_Dynamic_Trigger_Two_Layers_NoRA/Communication Preparation 2/Event Tigger Mechanism/Event trigger ==
  data: time input; E_norm output; trigger_flag output; info_trigger output; delta_xi_now input; beta_i output; delta_vi_now input; e_tilde input; info_prev input; beta_i_prev input
function [E_norm, trigger_flag, info_trigger, beta_i] = event_trigger_commu(time, delta_xi_now, delta_vi_now, e_tilde, info_prev, beta_i_prev)

dimension = 3;

commu_step = 0.01;
step_size = 0.01;

if mod(time,commu_step) == 0

    E_xi = delta_xi_now - info_prev(dimension * 0 + 1 : dimension * 1);
    E_vi = delta_vi_now - info_prev(dimension * 1 + 1 : dimension * 2);
    trigger_flag = 0;
    info_trigger = info_prev;
    
    Q_max = 3.0;
    A_tilde = 2.5;
    P_min = 0.4;
    Lambda_min = 2;
    C_i = 2* eye(3);
    Lambda_i = 2* eye(3);
    rho_2 = 0.3;
    rho_3 = 0.5;
    alpha_1 = 1;
    
    gamma_2 = 0.5;
    
    F_2 = norm(Q_max * A_tilde * C_i * E_vi)^2/2 + norm(Q_max * A_tilde * C_i * Lambda_i * E_xi)^2/2 + 5 * rho_2 * P_min * Lambda_min * A_tilde^2 * norm(E_xi)^2 - 3 * rho_2 * P_min * Lambda_min * norm(e_tilde)^2/4;
    
    % Trigger check
    if F_2 - gamma_2 * beta_i_prev >=0
        trigger_flag = 1;
        F_2 = - 3 * rho_2 * P_min * Lambda_min * norm(e_tilde)^2/4;
        info_trigger = [delta_xi_now; delta_vi_now];
    end
    
    % If we abandon the event triggered scheme
    % info_trigger = [delta_xi_now; delta_vi_now];
    
    E_norm = norm(info_trigger - [delta_xi_now; delta_vi_now]);
    
    beta_i_dot = - alpha_1 * beta_i_prev - F_2 + rho_3;
    
    beta_i = beta_i_prev + beta_i_dot * step_size;

else
    info_trigger = info_prev;
    E_norm = norm(info_trigger - [delta_xi_now; delta_vi_now]);
    trigger_flag = 0;
    beta_i = beta_i_prev;
end

end

== matlab function MVS_Dynamic_Trigger_Two_Layers_NoRA/Communication Preparation 2/Reference Filter/Adaptive filter/Nominal filter ==
  data: pos_ref input; u_i_nom output; vel_ref input; current_pos input; filter_error output
function [u_i_nom, filter_error]= nominal_filter(pos_ref, vel_ref, current_pos)

filter_error = current_pos - pos_ref;
k = 2 * eye(3);

u_i_nom = - k * filter_error + vel_ref;

end

== matlab function MVS_Dynamic_Trigger_Two_Layers_NoRA/High-Level Agent 2/Trajectory Planner/Achievability assurance/Nominal SMC ==
  data: delta_x input; u_restrict output; delta_v input; a_d input; delta_norm output
function [u_restrict, delta_norm] = slide_control(delta_x, delta_v, a_d)

c = 1 * eye(3);
lambda = 1 * eye(3);
r_1 = 1.5;        % Maximum difference
% r_2 = 0.5;
k_tilde = 2;

s = delta_v + lambda * delta_x;
delta_norm = norm(delta_x);

choice = 1;

switch choice
    case 1
        u_restrict = a_d - lambda * delta_v - c * s - k_tilde /(r_1^2 - norm(delta_x)^2) * delta_x;
    case 2
        u_restrict = a_d - lambda * delta_v - c * s - delta_x;
    case 3
        u_restrict = - lambda * delta_v - c * s - k_tilde * 3 * delta_x / (r_1^2 - norm(delta_x)^2);
    case 4
        u_restrict = - lambda * delta_v - c * s - k_tilde * delta_x;
end

%% Known physical acceleration
% u_restrict = a_d - lambda * delta_v - (r_1^2 - norm(s)^2) * c * s;
% u_restrict = a_d - lambda * delta_v - c * s - 2 * max(3 /(r_1^2 - norm(delta_x)^2), 1) * delta_x;
% u_restrict = a_d - lambda * delta_v - c * s - 2 * (r_1^2 - r_2^2) /(r_1^2 - norm(delta_x)^2) * delta_x;
% u_restrict = a_d - lambda * delta_v - c * s - delta_x;

%% Unknown physical acceleration
% u_restrict = - lambda * delta_v - c * s - 2 * 3 * delta_x / (r_1^2 - norm(delta_x)^2);
% u_restrict = - lambda * delta_v - c * s - 2 * delta_x;

end

== matlab function MVS_Dynamic_Trigger_Two_Layers_NoRA/High-Level Agent 2/Trajectory Planner/Cooperative tracking/Input compensator ==
  data: u_i_slide input; v_i input; u_i_actual output; Xi_i input; Xi_i_dot output
function [u_i_actual, Xi_i_dot] = input_compensator(u_i_slide, v_i, Xi_i)

%% Basic parameters
eta_1 = 10 * eye(3);
eta_2 = 0.5 * eye(3);
eta_3 = 6 * eye(3);
U_Mi = [2;2;1.5];

Xi_m = 5;

%% Preliminary compensation
v_Mi = [5;5;4];
control_step = 0.01;
v_up = v_Mi - v_i;
v_low = -v_Mi - v_i;
u_up = min(v_up/control_step, U_Mi);
u_low = max(v_low/control_step, -U_Mi);

%% Calculate the actual control input
u_i = u_i_slide - eta_3 * Xi_i;
u_i_actual = u_i;

for i = 1 : size(u_i_actual,1)
    if u_i(i) > u_up(i)
        u_i_actual(i) = u_up(i);
    elseif u_i(i) < u_low(i)
        u_i_actual(i) = u_low(i);
    end
end

u_tilde_i = u_i - u_i_actual;

if norm(Xi_i) < Xi_m
    Xi_i_dot = eta_1 * u_tilde_i - eta_2 * Xi_i;
else
    Xi_i_dot = eta_1 * u_tilde_i - eta_2 * Xi_i - norm(u_tilde_i)^2/norm(Xi_i)^2;
end

end

== matlab function MVS_Dynamic_Trigger_Two_Layers_NoRA/High-Level Agent 2/Trajectory Planner/Cooperative tracking/Nominal sliding mode controller ==
  data: u_i_slide output; e_tilde_xi input; e_tilde_vi input; delta_xi input; delta_vi input; acl_ref_agent input
function u_i_slide = nominal_sliding_controller(e_tilde_xi, e_tilde_vi, delta_xi, delta_vi, acl_ref_agent)

%% This is the nominal sliding mode controller for precise reference tracking

%% Basic parameters
C_i = 2 * eye(3);
Lambda_i = 2 * eye(3);

%% Controller
% Control input
S_tilde_i = e_tilde_vi + Lambda_i * e_tilde_xi;

u_i_slide = - C_i * S_tilde_i - Lambda_i * delta_vi - delta_xi + acl_ref_agent;

end

== matlab function MVS_Dynamic_Trigger_Two_Layers_NoRA/High-Level Agent 2/Trajectory Planner/Input compensator ==
  data: u_i_track input; u_i_restrict input; u_i output; delta_low_norm input
function u_i  = input_compensator(u_i_track, u_i_restrict, delta_low_norm)

%% Basic parameters
r_2 = 0.5;
r_3 = 0.8;

%% Calculate the actual control input
scenario = 2;

switch scenario
    case 1
        if delta_low_norm < r_2
            u_i = u_i_track;
        elseif delta_low_norm >= r_2 && delta_low_norm < r_3
            u_i = (r_3 - delta_low_norm)/(r_3 - r_2) * u_i_track + (delta_low_norm - r_2)/(r_3 - r_2) * u_i_restrict;
        else
            u_i = u_i_restrict;
        end

    case 2
        u_i = u_i_track;
end

end

== matlab function MVS_Dynamic_Trigger_Two_Layers_NoRA/High-Level Agent 1/Trajectory Planner/Achievability assurance/Input compensator ==
  data: u_i_restrict input; v_i input; u_i_actual output; Xi_i input; Xi_i_dot output
function [u_i_actual, Xi_i_dot] = input_compensator(u_i_restrict, v_i, Xi_i)

%% Basic parameters
eta_1 = 10 * eye(3);
eta_2 = 0.5 * eye(3);
eta_3 = 6 * eye(3);
U_Mi = [2;2;1.5];

Xi_m = 5;

%% Preliminary compensation
v_Mi = [5;5;4];
control_step = 0.01;
v_up = v_Mi - v_i;
v_low = -v_Mi - v_i;
u_up = min(v_up/control_step, U_Mi);
u_low = max(v_low/control_step, -U_Mi);

%% Calculate the actual control input
u_i = u_i_restrict - eta_3 * Xi_i;
u_i_actual = u_i;

for i = 1 : size(u_i_actual,1)
    if u_i(i) > u_up(i)
        u_i_actual(i) = u_up(i);
    elseif u_i(i) < u_low(i)
        u_i_actual(i) = u_low(i);
    end
end

u_tilde_i = u_i - u_i_actual;

if norm(Xi_i) < Xi_m
    Xi_i_dot = eta_1 * u_tilde_i - eta_2 * Xi_i;
else
    Xi_i_dot = eta_1 * u_tilde_i - eta_2 * Xi_i - norm(u_tilde_i)^2/norm(Xi_i)^2;
end

end

== matlab function MVS_Dynamic_Trigger_Two_Layers_NoRA/Communication Preparation 4/Event Tigger Mechanism/Event trigger ==
  data: time input; E_norm output; trigger_flag output; info_trigger output; delta_xi_now input; beta_i output; delta_vi_now input; e_tilde input; info_prev input; beta_i_prev input
function [E_norm, trigger_flag, info_trigger, beta_i] = event_trigger_commu(time, delta_xi_now, delta_vi_now, e_tilde, info_prev, beta_i_prev)

dimension = 3;

commu_step = 0.01;
step_size = 0.01;

if mod(time,commu_step) == 0

    E_xi = delta_xi_now - info_prev(dimension * 0 + 1 : dimension * 1);
    E_vi = delta_vi_now - info_prev(dimension * 1 + 1 : dimension * 2);
    trigger_flag = 0;
    info_trigger = info_prev;
    
    Q_max = 3.0;
    A_tilde = 2.5;
    P_min = 0.4;
    Lambda_min = 2;
    C_i = 2* eye(3);
    Lambda_i = 2* eye(3);
    rho_2 = 0.3;
    rho_3 = 0.5;
    alpha_1 = 1;
    
    gamma_2 = 0.5;
    
    F_2 = norm(Q_max * A_tilde * C_i * E_vi)^2/2 + norm(Q_max * A_tilde * C_i * Lambda_i * E_xi)^2/2 + 5 * rho_2 * P_min * Lambda_min * A_tilde^2 * norm(E_xi)^2 - 3 * rho_2 * P_min * Lambda_min * norm(e_tilde)^2/4;
    
    % Trigger check
    if F_2 - gamma_2 * beta_i_prev >=0
        trigger_flag = 1;
        F_2 = - 3 * rho_2 * P_min * Lambda_min * norm(e_tilde)^2/4;
        info_trigger = [delta_xi_now; delta_vi_now];
    end
    
    % If we abandon the event triggered scheme
    % info_trigger = [delta_xi_now; delta_vi_now];
    
    E_norm = norm(info_trigger - [delta_xi_now; delta_vi_now]);
    
    beta_i_dot = - alpha_1 * beta_i_prev - F_2 + rho_3;
    
    beta_i = beta_i_prev + beta_i_dot * step_size;

else
    info_trigger = info_prev;
    E_norm = norm(info_trigger - [delta_xi_now; delta_vi_now]);
    trigger_flag = 0;
    beta_i = beta_i_prev;
end

end

== matlab function MVS_Dynamic_Trigger_Two_Layers_NoRA/Communication Preparation 4/Reference Filter/Adaptive filter/Input compensator ==
  data: u_i_nom input; u_i output; Xi_i input; Xi_i_dot output
function [u_i, Xi_i_dot] = input_compensator(u_i_nom, Xi_i)

%% Basic parameters
eta_1 = 10 * eye(3);
eta_2 = 0.5 * eye(3);
eta_3 = 6 * eye(3);
v_Mi = [5;5;4];

Xi_m = 5;

%% Calculate the actual control input
u_i = u_i_nom - eta_3 * Xi_i;
u_i_actual = u_i;

u_up = v_Mi;
u_low = - v_Mi;

for i = 1 : size(u_i_actual,1)
    if u_i(i) > u_up(i)
        u_i_actual(i) = u_up(i);
    elseif u_i(i) < u_low(i)
        u_i_actual(i) = u_low(i);
    end
end

u_tilde_i = u_i - u_i_actual;

if norm(Xi_i) < Xi_m
    Xi_i_dot = eta_1 * u_tilde_i - eta_2 * Xi_i;
else
    Xi_i_dot = eta_1 * u_tilde_i - eta_2 * Xi_i - norm(u_tilde_i)^2/norm(Xi_i)^2;
end

% Xi_i_dot = [0;0;0];

end
